simulink model "problem7"  (R2020b)
settings: Solver=VariableStepAuto  StartTime=0.0  StopTime=10.0  RelTol=1e-3
settings Model: Creator=admin  LastModifiedBy=admin

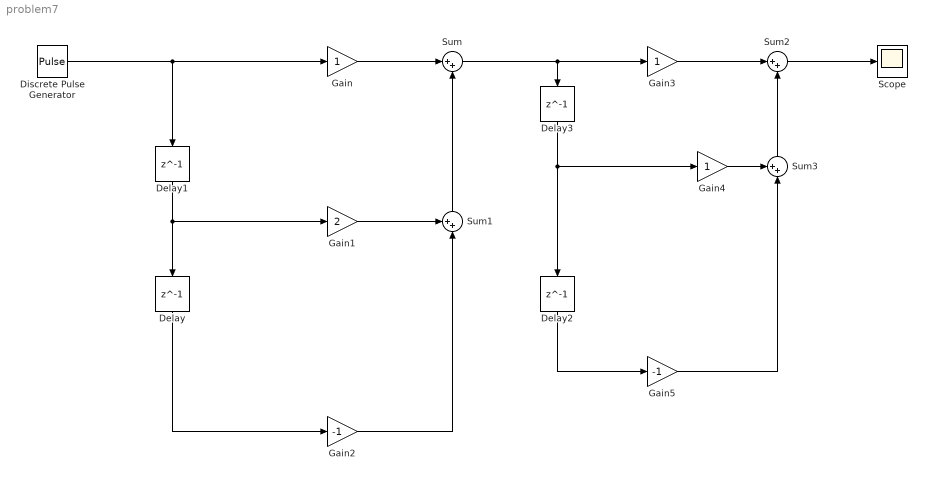
== system problem7 ==
  Delay{,1..3} (4 alike) : Delay  DelayLength=1
  Discrete Pulse Generator : DiscretePulseGenerator  Period=10  PulseWidth=5
  Gain : Gain
  Gain1 : Gain  Gain=2
  Gain2 : Gain  Gain=-1
  Gain3 : Gain
  Gain4 : Gain
  Gain5 : Gain  Gain=-1
  Scope : Scope
  Sum : Sum  Inputs=|++
  Sum1 : Sum  Inputs=++|
  Sum2 : Sum  Inputs=|++
  Sum3 : Sum  Inputs=++|
  wires:
  Delay2/1 -> Gain5/1
  Sum2/1 -> Scope/1
  Gain5/1 -> Sum3/2
  Delay1/1 -> Gain1/1, Delay/1
  Gain4/1 -> Sum3/1
  Delay3/1 -> Gain4/1, Delay2/1
  Sum/1 -> Gain3/1, Delay3/1
  Sum1/1 -> Sum/2
  Gain1/1 -> Sum1/1
  Sum3/1 -> Sum2/2
  Gain/1 -> Sum/1
  Discrete Pulse Generator/1 -> Gain/1, Delay1/1
  Gain3/1 -> Sum2/1
  Delay/1 -> Gain2/1
  Gain2/1 -> Sum1/2
